simulink model "angular_control"  (R2023a)
settings: Solver=ode45  StartTime=0.0  StopTime=6179  RelTol=1e-3  EnableMultiTasking=on
undefined symbols (not defined in the file): ang_ref_value, est_on_off, momentum_dyn_on, ref_change1, ref_change2
libraries: components_lib x7, simulink x1
settings Model: Creator=krage  LastModifiedBy=jacobel-omar
settings SolverCC: AlgebraicLoopSolver=TrustRegion
settings DataIOCC: LimitDataPoints=on  SaveFormat=Array  SignalLoggingSaveFormat=ModelDataLogs  ReturnWorkspaceOutputs=off
settings OptimizationCC: InitFltsAndDblsToZero=on  LifeSpan=inf
settings DebuggingCC: SaveWithParameterizedLinksMsg=none  CheckSSInitialOutputMsg=off  UnderspecifiedInitializationDetection=Classic  MergeDetectMultiDrivingBlocksExec=none  SignalResolutionControl=TryResolveAllWithWarning  SolverPrmCheckMsg=warning  MultiTaskDSMMsg=warning  MultiTaskCondExecSysMsg=none  FcnCallInpInsideContextMsg=warning  UnconnectedInputMsg=warning  UnconnectedOutputMsg=warning  UnconnectedLineMsg=warning  SFUnexpectedBacktrackingDiag=warning  SFNoUnconditionalDefaultTransitionDiag=warning  SFExecutionAtInitializationDiag=none  ArithmeticOperatorsInVariantConditions=warning
settings HardwareCC: ProdBitPerPointer=32  ProdBitPerSizeT=32  ProdBitPerPtrDiffT=32  ProdLargestAtomicFloat=None  ProdIntDivRoundTo=Undefined  ProdEndianess=Unspecified  ProdWordSize=32  ProdHWDeviceType=32-bit Generic
settings ModelReferenceCC: PropagateSignalLabelsOutOfModel=off
settings CodeAppCC: StateflowObjectComments=on
settings GRTTargetCC: TargetFcnLib=ansi_tfl_tmw.mat  TargetLangStandard=C89/C90 (ANSI)  CombineOutputUpdateFcns=off  GRTInterface=on
settings ConfigComp: CovMetricSettings=dw  CovSaveCumulativeToWorkspaceVar=on  CovSaveSingleToWorkspaceVar=on

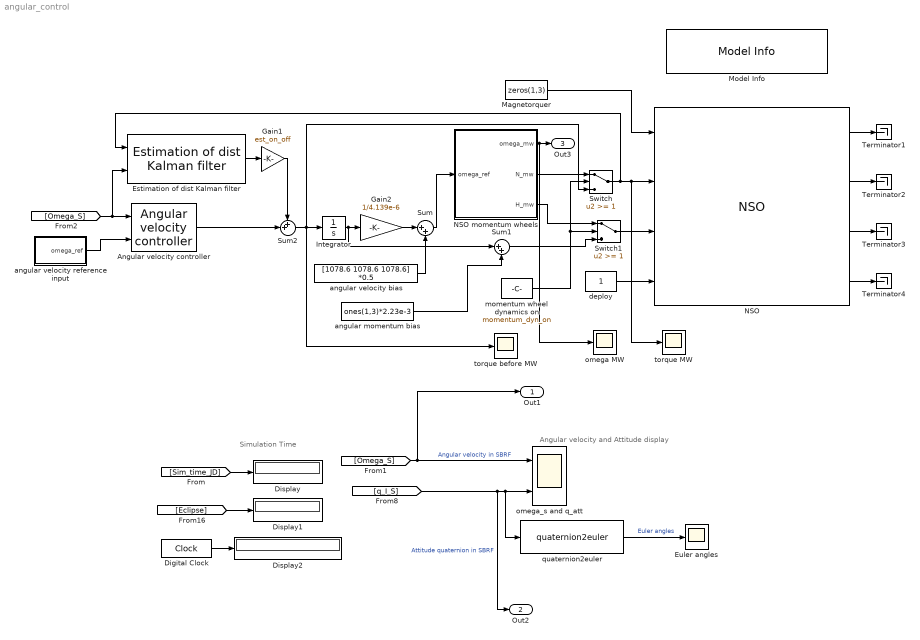
== system angular_control ==
  note: Simulation Time
  note: Angular velocity and Attitude display
  Angular velocity controller : components_lib/ACS/Controllers/Angular velocity  controller  ang_file_name=ang_control_config
  Digital Clock : DigitalClock
  Display : Display
  Display1 : Display
  Display2 : Display
  Estimation of dist Kalman filter : components_lib/ACS/Controllers/Estimation of dist Kalman filter  ang_file_name=ang_estimation_config
  Euler angles : Scope
  Gain1 : Gain  Gain=est_on_off
  Gain2 : Gain  Gain=1/4.139e-6
  Integrator : Integrator
  Magnetorquer : Constant  Value=zeros(1,3)
  Model Info : simulink/Model-Wide Utilities/Model Info  Frame=on  DisplayStringWithTags=|  HorizontalTextAlignment=Center  LeftAlignmentValue=0.5
      | sun to eclipse : 2452315.560376
      | 32 sec. before : 2452315.56
      | eclipse to sun : 2452315.513363
  NSO : components_lib/NSO  Tag=AAUSAT-II Model  Description=AAUSAT-II Model  r_com_s=[0.05 0.05 0.15]  sat_temp_start=0  r_com_s_deployed=[0.05 0.05 0.125]  mass_sc=3  Dim=[0.1 0.1 0.3]  inertia_c=[25 25 5]/1e3  inertia_d=inertial_matrix  init_jd=2452315.56  q_s_c=[0 0 0 1]  q_init_s_i=ang_attitude  w_init_s=init_ang_vel  Cd=cd_value  rho=air_density  enable_sensor_emulation=off  alb_emu_enabled=off  enable_dist=on
      link override Inertia deployed2: Value=[0 0 0]
  NSO momentum wheels : Subsystem  AncestorBlock=components_lib/Actuator Emulation/NSO momentum wheels  mask{w_mw_i=[1078.6 1078.6 1078.6] *0.5}
      mask prompts: w_mw_i "Initial Angular Velocity"
  Sum : Sum  Inputs=|++
  Sum1 : Sum  Inputs=|++
  Sum2 : Sum  Inputs=++|
  Switch : Switch  Threshold=1  SaturateOnIntegerOverflow=off  InputSameDT=off
  Switch1 : Switch  Threshold=1  SaturateOnIntegerOverflow=off  InputSameDT=off
  Terminator{1..4} (4 alike) : Terminator
  angular momentum bias : Constant  Value=ones(1,3)*2.23e-3
  angular velocity reference input : Subsystem
  angular velocity bias : Constant  Value=[1078.6 1078.6 1078.6] *0.5
  deploy : Constant
  momentum wheel dynamics on : Constant  Value=momentum_dyn_on
  omega MW : Scope
  omega_s and q_att : Scope  NumInputPorts=2
  quaternion2euler : components_lib/Math utilities/Quaternion operations/quaternion2euler  SystemSampleTime=-1  VariantActivationTime=update diagram  Latency=0  AutoFrameSizeCalculation=off
  torque MW : Scope
  torque before MW : Scope
  Out1 : Outport
  Out2 : Outport  Port=2
  Out3 : Outport  Port=3
  wires:
  [q_I_S] -> omega_s and q_att/2, quaternion2euler/1, Out2/1  "Attitude quaternion in SBRF"
  quaternion2euler/1 -> Euler angles/1  "Euler angles"
  [Sim_time_JD] -> Display/1
  [Eclipse] -> Display1/1
  Digital Clock/1 -> Display2/1
  deploy/1 -> NSO/4
  [Omega_S] -> Angular velocity controller/1, Estimation of dist Kalman filter/2
  NSO momentum wheels/2(N_mw) -> Switch/1
  Gain2/1 -> Sum/1
  Sum/1 -> NSO momentum wheels/1(omega_ref)
  angular velocity bias/1 -> Sum/2
  Integrator/1 -> Gain2/1, Sum1/1
  [Omega_S] -> omega_s and q_att/1, Out1/1  "Angular velocity in SBRF"
  Estimation of dist Kalman filter/1 -> Gain1/1
  Angular velocity controller/1 -> Sum2/2
  Sum2/1 -> Integrator/1, Switch/3, torque before MW/1
  Magnetorquer/1 -> NSO/1
  Gain1/1 -> Sum2/1
  angular velocity reference input/1(omega_ref) -> Angular velocity controller/2
  NSO momentum wheels/1(omega_mw) -> Out3/1, omega MW/1
  NSO/1 -> Terminator1/1
  NSO/2 -> Terminator2/1
  NSO/3 -> Terminator3/1
  NSO/4 -> Terminator4/1
  Switch1/1 -> NSO/3
  Switch/1 -> Estimation of dist Kalman filter/1, NSO/2, torque MW/1
  NSO momentum wheels/3(H_mw) -> Switch1/1
  momentum wheel dynamics on/1 -> Switch/2, Switch1/2
  Sum1/1 -> Switch1/3
  angular momentum bias/1 -> Sum1/2

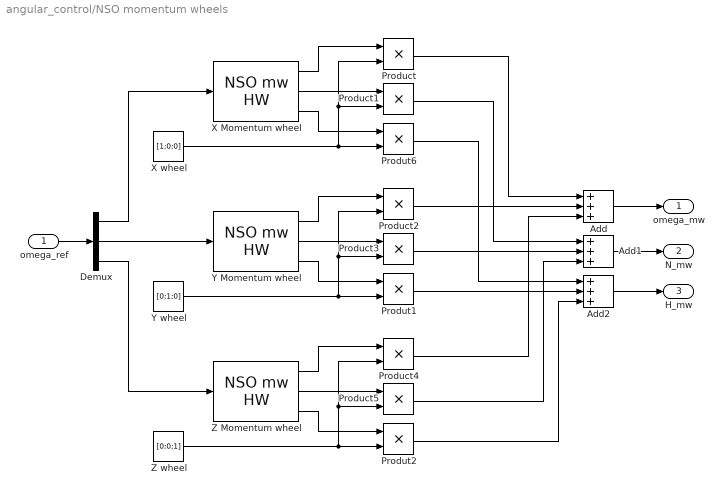
== system angular_control/NSO momentum wheels ==
  omega_ref : Inport
  Add : Sum  Inputs=+++
  Add1 : Sum  Inputs=+++
  Add2 : Sum  Inputs=+++
  Demux : Demux  Outputs=3
  Product{,1..5} (6 alike) : Product  RndMeth=Zero
  Produt1 : Product  RndMeth=Zero
  Produt2 : Product  RndMeth=Zero
  Produt6 : Product  RndMeth=Zero
  X Momentum wheel : components_lib/Actuator Emulation/NSO mw HW  C_p=0.01  C_i=0.001  w_mw_init=w_mw_i(1)
  X wheel : Constant  Value=[1;0;0]
  Y Momentum wheel : components_lib/Actuator Emulation/NSO mw HW  C_p=0.01  C_i=0.001  w_mw_init=w_mw_i(2)
  Y wheel : Constant  Value=[0;1;0]
  Z Momentum wheel : components_lib/Actuator Emulation/NSO mw HW  C_p=0.01  C_i=0.001  w_mw_init=w_mw_i(3)
  Z wheel : Constant  Value=[0;0;1]
  omega_mw : Outport  PortDimensions=3
  N_mw : Outport  Port=2  PortDimensions=3
  H_mw : Outport  Port=3  PortDimensions=3
  wires:
  Demux/2 -> Y Momentum wheel/1
  Demux/3 -> Z Momentum wheel/1
  Demux/1 -> X Momentum wheel/1
  omega_ref/1 -> Demux/1
  Product4/1 -> Add/3
  Product5/1 -> Add1/3
  Produt2/1 -> Add2/3
  Z Momentum wheel/2 -> Product5/1
  Z Momentum wheel/1 -> Product4/1
  Z Momentum wheel/3 -> Produt2/1
  Z wheel/1 -> Produt2/2, Product5/2, Product4/2
  Produt1/1 -> Add2/2
  Product3/1 -> Add1/2
  Product2/1 -> Add/2
  Y Momentum wheel/2 -> Product3/1
  Y Momentum wheel/1 -> Product2/1
  Y Momentum wheel/3 -> Produt1/1
  Y wheel/1 -> Produt1/2, Product3/2, Product2/2
  X Momentum wheel/2 -> Product1/1
  X Momentum wheel/1 -> Product/1
  X Momentum wheel/3 -> Produt6/1
  Add/1 -> omega_mw/1
  X wheel/1 -> Produt6/2, Product1/2, Product/2
  Add1/1 -> N_mw/1
  Product/1 -> Add/1
  Product1/1 -> Add1/1
  Add2/1 -> H_mw/1
  Produt6/1 -> Add2/1

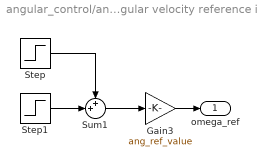
== system angular_control/angular velocity reference input ==
  Gain3 : Gain  Gain=ang_ref_value
  Step : Step  Time=ref_change1  SampleTime=0
  Step1 : Step  Time=ref_change2  After=-1  SampleTime=0
  Sum1 : Sum  Inputs=++|
  omega_ref : Outport
  wires:
  Step1/1 -> Sum1/2
  Step/1 -> Sum1/1
  Sum1/1 -> Gain3/1
  Gain3/1 -> omega_ref/1
